simulink model "roketProje2220x2810x29"  (R2024a)
settings: Solver=ode4  StartTime=0.0  StopTime=3.5  FixedStep=0.01  RelTol=1e-3
undefined symbols (not defined in the file): magnitude
settings Model: Creator=esrademir  LastModifiedBy=LENOVO
settings OptimizationCC: ReuseModelBlockBuffer=off
settings RTWCC: GPUComputeCapability=3.5

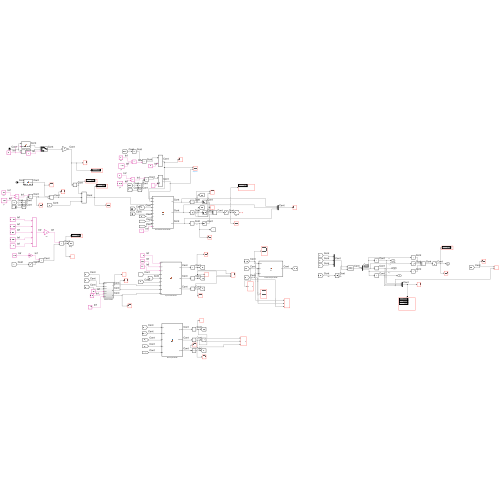
[thumbnail: Simulink's stored preview of the top-level diagram]
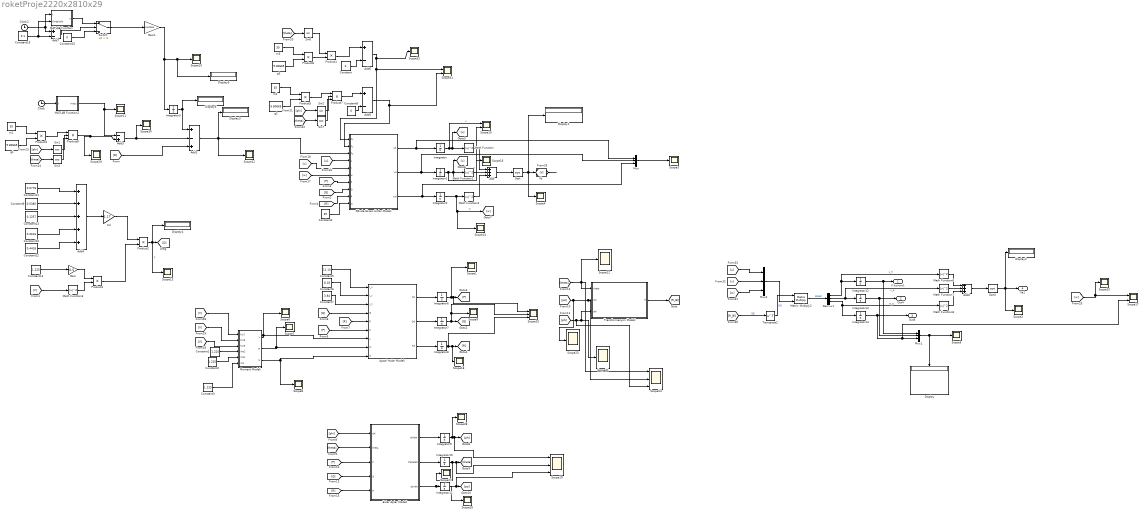
== system roketProje2220x2810x29 ==
  Add : Sum  Inputs=+++
  Add1 : Sum  Inputs=+-+
  Add2 : Sum  Inputs=+++
  Add3 : Sum  Inputs=-+
  Add4 : Sum  Inputs=+++++
  Add5 : Sum  Inputs=+-
  Add6 : Sum  Inputs=+-
  Add7 : Sum  Inputs=+-
  Açısal Hızlar Modeli : MATLAB Function  TreatAsAtomicUnit=on
  Cd : Gain  Gain=1.17
  Clock : Clock
  Clock2 : Clock
  Constant : Constant  Value=0
  Constant{1..3,14} (4 alike) : Constant  Value=1.225
  Constant10 : Constant  Value=0.0616
  Constant11 : Constant  Value=0.0778
  Constant12 : Constant  Value=0.4418
  Constant13 : Constant  Value=0.1257
  Constant15 : Constant  Value=0
  Constant16 : Constant  Value=0.1
  Constant4 : Constant  Value=35
  Constant5 : Constant  Value=11.13
  Constant6 : Constant  Value=8.18
  Constant7 : Constant  Value=3.84
  Constant8 : Constant  Value=0
  Constant9 : Constant  Value=0.0380
  Demux1 : Demux  Outputs=3
  Display{,1..6} (7 alike) : Display
  Euler Açılar Modeli : MATLAB Function  TreatAsAtomicUnit=on
  Gain : Gain  Gain=0.5
  Gain1 : Gain  Gain=3.52250
  Gövde Eksen Hızlar Modeli : MATLAB Function  TreatAsAtomicUnit=on
  Integrator{,1..3,6..10,12..13} (11 alike) : Integrator
  Integrator11 : Integrator  InitialCondition=1.5
  Integrator14 : Integrator  InitialCondition=9
  MATLAB Function : MATLAB Function  TreatAsAtomicUnit=on
  MATLAB Function2 : MATLAB Function  TreatAsAtomicUnit=on
  Math Function{,1..3,6..8} (7 alike) : Math  Operator=magnitude^2
  Matrix Multiply2 : Product  Multiplication=Matrix(*)
  Moment Modeli : Subsystem
  Mux : Mux  Inputs=3
  Mux1 : Mux  Inputs=3
  Mux2 : Mux  Inputs=3
  Product{1..6} (6 alike) : Product
  Product7 : Product  Inputs=3
  Product8 : Product  Inputs=3
  Scope{1..14,16,18,20..23,26..30,32} (26 alike) : Scope
  Scope15 : Scope  NumInputPorts=2
  Scope17 : Scope  NumInputPorts=2
  Scope19 : Scope  NumInputPorts=3
  Scope24 : Scope  NumInputPorts=3
  Scope25 : Scope  NumInputPorts=3
  Scope31 : Scope  NumInputPorts=2
  Sin1 : Trigonometry  Operator=cos
  Sin2 : Trigonometry
  Sin3 : Trigonometry  Operator=cos
  Sin6 : Trigonometry
  Sin7 : Trigonometry  Operator=cos
  Sqrt : Sqrt
  Sqrt2 : Sqrt
  Switch : Switch  Criteria=u2 > Threshold  SaturateOnIntegerOverflow=off  InputSameDT=off
  Transformasyon Modeli : MATLAB Function  TreatAsAtomicUnit=on
  Transpose2 : Math  Operator=transpose
  g1 : Constant  Value=9.80665
  g2 : Constant  Value=9.80665
  g3 : Constant  Value=9.80665
  m1 : Constant  Value=35
  m2 : Constant  Value=35
  m3 : Constant  Value=35
  X konum1 : Outport
  Out4 : Outport  Port=2
  Out5 : Outport  Port=3
  Ve1 : Outport  Port=4
  wires:
  Constant/1 -> Add6/2
  Gövde Eksen Hızlar Modeli/2(vd) -> Mux/2, Integrator1/1
  Math Function7/1 -> Add2/2
  [phi] -> Sin2/1
  Constant7/1 -> Açısal Hızlar Modeli/3(I_z)
  [w] -> Mux2/3
  Constant5/1 -> Açısal Hızlar Modeli/1(I_x)
  Product5/1 -> Product7/1
  Constant8/1 -> Add5/2
  Demux1/3 -> Integrator14/1, Math Function8/1  "w_e"
  [R] -> Euler Açılar Modeli/5(R)
  Add6/1 -> Scope32/1, Gövde Eksen Hızlar Modeli/1(Fx), Scope31/1
  Clock/1 -> MATLAB Function2/1(t)
  Product6/1 -> Product1/2
  [phi] -> Scope24/3, Scope21/1, Transformasyon Modeli/3(phi)
  Matrix Multiply2/1 -> Demux1/1  "atalet"
  MATLAB Function/1(T) -> Switch/1
  [v] -> Mux2/2
  [theta] -> Euler Açılar Modeli/2(theta)
  Product1/1 -> Add6/1
  [theta] -> Sin6/1
  Sin3/1 -> Product8/3
  [P] -> Açısal Hızlar Modeli/6(P)
  Integrator12/1 -> X konum1/1, Mux1/1
  m3/1 -> Product6/1
  [theta] -> Sin3/1
  Sin7/1 -> Product7/3
  g2/1 -> Product5/2
  MATLAB Function2/1(mass) -> Scope11/1, Add3/1
  [theta] -> Sin7/1
  Integrator13/1 -> Out4/1, Mux1/2
  [Q] -> Euler Açılar Modeli/4(Q)
  Add5/1 -> Scope31/2, Gövde Eksen Hızlar Modeli/2(Fy)
  Integrator/1 -> Scope15/1, [u], Math Function/1  "u"
  Constant13/1 -> Add4/3
  Mux/1 -> Scope3/1
  Math Function8/1 -> Add2/3
  g3/1 -> Product6/2
  Mux1/1 -> Scope5/1, Display/1
  Moment Modeli/3(N) -> Açısal Hızlar Modeli/9(N), Scope8/1
  [Q] -> Açısal Hızlar Modeli/4(Q)
  Integrator9/1 -> Scope28/1, Scope19/1, [phi]
  Gain/1 -> Product4/1
  [u] -> Mux2/1
  Constant2/1 -> Moment Modeli/5(rho1)
  [w] -> Gövde Eksen Hızlar Modeli/6(w)
  Math Function3/1 -> Product4/2
  [R] -> Gövde Eksen Hızlar Modeli/9(R)
  [P] -> Gövde Eksen Hızlar Modeli/7(P)
  Demux1/2 -> Math Function7/1, Integrator13/1  "v_e"
  Math Function6/1 -> Add2/1
  [psi] -> Scope23/1, Scope24/2, Transformasyon Modeli/2(psi)
  [D] -> Add1/3
  Mux2/1 -> Matrix Multiply2/2
  Math Function/1 -> Add/1
  Integrator7/1 -> Scope25/2, Scope9/1, [Q]
  Integrator3/1 -> Display6/1, Add1/1
  Constant12/1 -> Add4/5
  Product4/1 -> Product2/2
  Constant16/1 -> MATLAB Function/2(threshold), Add7/2
  [V] -> Math Function3/1
  Euler Açılar Modeli/3(psidot) -> Scope26/1, Integrator11/1
  Integrator14/1 -> Out5/1, Scope17/2, Mux1/3
  Constant11/1 -> Add4/1
  Açısal Hızlar Modeli/1(Pd) -> Integrator6/1
  Sin1/1 -> Product8/2
  Integrator8/1 -> Scope25/3, Scope18/1, [R]
  Integrator6/1 -> Scope25/1, [P], Scope1/1
  Constant10/1 -> Add4/4
  Product2/1 -> Scope13/1, Display4/1, [D]  "F"
  Constant9/1 -> Add4/2
  Add4/1 -> Cd/1
  Add/1 -> Sqrt/1
  [P] -> Euler Açılar Modeli/3(P)
  m2/1 -> Product5/1
  Integrator1/1 -> Scope15/2, [v], Scope16/1, Math Function1/1  "v"
  Math Function1/1 -> Add/2
  Moment Modeli/1(L) -> Açısal Hızlar Modeli/7(L), Scope6/1
  Moment Modeli/2(M) -> Scope7/1, Açısal Hızlar Modeli/8(M)
  [theta] -> Scope24/1, Scope22/1, Transformasyon Modeli/1(theta)
  [R_BI] -> Transpose2/1  "I2B"
  Add7/1 -> Switch/2
  [phi] -> Sin1/1
  [V] -> Moment Modeli/2(hız8)
  Transformasyon Modeli/1(R) -> [R_BI]
  Product3/1 -> Product8/1
  Clock2/1 -> MATLAB Function/1(t), Add7/1
  [v] -> Gövde Eksen Hızlar Modeli/5(v)
  Gövde Eksen Hızlar Modeli/3(wd) -> Mux/3, Integrator2/1
  [w] -> Scope20/1, Scope17/1
  Açısal Hızlar Modeli/3(Rd) -> Integrator8/1
  Add2/1 -> Sqrt2/1
  Constant1/1 -> Moment Modeli/4(rho2)
  [Q] -> Gövde Eksen Hızlar Modeli/8(Q)
  Açısal Hızlar Modeli/2(Qd) -> Integrator7/1
  Integrator11/1 -> Scope19/3, [psi]
  Sin2/1 -> Product7/2
  Gain1/1 -> Integrator3/1, Display5/1, Scope10/1
  [V] -> Moment Modeli/3(hız9)
  Add1/1 -> Gövde Eksen Hızlar Modeli/3(Fz), Scope12/1, Display3/1
  Euler Açılar Modeli/1(phidot) -> Integrator9/1
  Integrator2/1 -> Scope14/1, [w], Math Function2/1  "w"
  [phi] -> Euler Açılar Modeli/1(phi)
  Constant3/1 -> Moment Modeli/6(rho)
  Product7/1 -> Add5/1
  Integrator10/1 -> Scope27/1, Scope19/2, [theta]
  Demux1/1 -> Math Function6/1, Integrator12/1  "u_e"
  Sin6/1 -> Product1/1
  Gövde Eksen Hızlar Modeli/1(ud) -> Mux/1, Integrator/1
  Constant6/1 -> Açısal Hızlar Modeli/2(I_y)
  Add3/1 -> Scope30/1, Add1/2
  Sqrt/1 -> Display1/1, [V], Scope4/1
  Constant15/1 -> Switch/3
  m1/1 -> Product3/1
  Constant14/1 -> Gain/1
  Math Function2/1 -> Add/3
  [R] -> Açısal Hızlar Modeli/5(R)
  [u] -> Gövde Eksen Hızlar Modeli/4(u)
  Cd/1 -> Product2/1
  Product8/1 -> Add3/2, Scope29/1
  Constant4/1 -> Gövde Eksen Hızlar Modeli/10(m)
  g1/1 -> Product3/2
  [V] -> Moment Modeli/1(hız7)
  Sqrt2/1 -> Ve1/1, Scope2/1, Display2/1
  Transpose2/1 -> Matrix Multiply2/1  "B2I"
  Switch/1 -> Gain1/1
  Euler Açılar Modeli/2(thetadot) -> Integrator10/1
  [V] -> ?

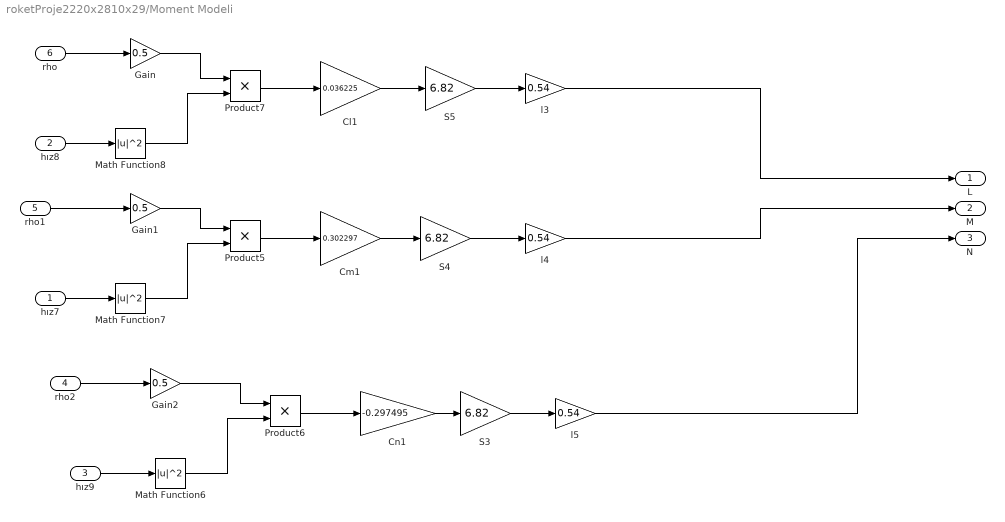
== system roketProje2220x2810x29/Moment Modeli ==
  hız7 : Inport
  hız8 : Inport  Port=2
  hız9 : Inport  Port=3
  rho2 : Inport  Port=4
  rho1 : Inport  Port=5
  rho : Inport  Port=6
  Cl1 : Gain  Gain=0.036225
  Cm1 : Gain  Gain=0.302297
  Cn1 : Gain  Gain=-0.297495
  Gain : Gain  Gain=0.5
  Gain1 : Gain  Gain=0.5
  Gain2 : Gain  Gain=0.5
  Math Function6 : Math  Operator=magnitude^2
  Math Function7 : Math  Operator=magnitude^2
  Math Function8 : Math  Operator=magnitude^2
  Product5 : Product
  Product6 : Product
  Product7 : Product
  S3 : Gain  Gain=6.82
  S4 : Gain  Gain=6.82
  S5 : Gain  Gain=6.82
  l3 : Gain  Gain=0.54
  l4 : Gain  Gain=0.54
  l5 : Gain  Gain=0.54
  L : Outport
  M : Outport  Port=2
  N : Outport  Port=3
  wires:
  S5/1 -> l3/1
  Product5/1 -> Cm1/1
  Product7/1 -> Cl1/1
  hız8/1 -> Math Function8/1
  Math Function7/1 -> Product5/2
  hız7/1 -> Math Function7/1
  S3/1 -> l5/1
  Math Function6/1 -> Product6/2
  rho1/1 -> Gain1/1
  Cl1/1 -> S5/1
  Cm1/1 -> S4/1
  Cn1/1 -> S3/1
  hız9/1 -> Math Function6/1
  Product6/1 -> Cn1/1
  Math Function8/1 -> Product7/2
  l5/1 -> N/1
  Gain2/1 -> Product6/1
  S4/1 -> l4/1
  Gain/1 -> Product7/1
  Gain1/1 -> Product5/1
  rho/1 -> Gain/1
  rho2/1 -> Gain2/1
  l3/1 -> L/1
  l4/1 -> M/1

== matlab function roketProje2220x2810x29/Açısal Hızlar Modeli ==
  data: I_x input; I_y input; I_z input; Q input; Pd output; R input; P input; L input; M input; N input; Qd output; Rd output
function [Pd, Qd, Rd] = fcn(I_x, I_y, I_z, Q, R, P, L, M, N)

Pd = Q*R*((I_x-I_z)/I_x)+L/I_x;
Qd = P*R*((I_z-I_x)/I_y)+M/I_y;
Rd = P*Q*((I_x-I_y)/I_z)+N/I_z;

 Qd=0;
Rd=0;
end

== matlab function roketProje2220x2810x29/Euler Açılar Modeli ==
  data: phi input; theta input; phidot output; P input; Q input; R input; thetadot output; psidot output
function [ phidot,  thetadot,  psidot] = fcn( phi, theta, P, Q, R)

A = (1/cos(theta))*[cos(theta) sin(phi)*sin(phi) cos(phi)*sin(phi);...
0 cos(phi)*cos(theta) sin(phi)*cos(theta);...
0  sin(phi) cos(phi)]*[P;Q;R];

phidot = A(1);
thetadot = A(2);
psidot = A(3);

== matlab function roketProje2220x2810x29/Gövde Eksen Hızlar Modeli ==
  data: Fx input; Fy input; Fz input; u input; ud output; v input; w input; P input; Q input; R input; vd output; wd output; m input
function [ud, vd, wd] = fcn(Fx, Fy, Fz, u, v, w, P, Q, R, m)

ud = (Fx/m)-w*Q+v*R;
vd = (Fy/m)-u*R+w*P;
wd = (Fz/m)-v*P+u*Q;

end

== matlab function roketProje2220x2810x29/MATLAB Function ==
  data: t input; T output; threshold input
function T = calculateThrust(t,threshold)
    if t >= threshold
        P = calculatePressure(t);
        T = fcn(P);
    else
        T = 0;
    end
end

function P = calculatePressure(t)
    % Denklemi hesapla
    P = 1000000 + 715*(t^2) - 213150*t;
end

function T = fcn(P)
    A = 0.0000956;
    T = A*P*(3.282*(1-(101000/P)^(0.4/1.4)))^(1/2);
end

== matlab function roketProje2220x2810x29/MATLAB Function2 ==
  data: t input; mass output
function mass = mass_over_time(t)
    % Zamanla değişen kütle hesaplama
    initial_mass = 0;  % Başlangıç kütlesi
    final_mass = 22.06496;  % Son kütle
    total_time = 3.065;  % Toplam süre

    if t <= total_time
        mass = initial_mass + (final_mass - initial_mass) * (t / total_time);
    else
        mass = final_mass;
    end

== matlab function roketProje2220x2810x29/Transformasyon Modeli ==
  data: theta input; psi input; phi input; R output
function R  = fcn(theta, psi, phi)    

R = [cos(theta)*cos(psi)  cos(theta)*sin(psi)  -sin(theta);...
     sin(phi)*sin(theta)*cos(psi)-cos(phi)*sin(psi)  sin(phi)*sin(theta)*sin(psi)+cos(theta)*cos(psi)  sin(phi)*cos(theta);...
     cos(phi)*sin(theta)*cos(psi)+sin(phi)*sin(psi)  cos(phi)*sin(theta)*sin(psi)-sin(phi)*cos(psi)  cos(phi)*cos(theta)];
